simulink model "mtv1_with_slosh"  (R2014b)
settings: Solver=ode4  SolverMode=SingleTasking  StartTime=0.0  StopTime=sim_stop_time  FixedStep=sim_time_step_size  RelTol=1e-3
PreLoadFcn:
  | nimbus_bus_all;
  | mtv_bus_all;
undefined symbols (not defined in the file or in its folder): csc_egt_egc_thruster, csc_egt_egc_thruster_lib, csc_eom_six_dof_integration_fwdeuler, csc_eom_six_dof_integration_lib, csc_rigid_body_dynamics, csc_rigid_body_dynamics_lib, csc_sim_mtv_simulation, csc_sim_mtv_simulation_lib, csc_thl_thrusters_mtv, csc_thl_thrusters_mtv_lib, csci_gsse_mtv, csci_gsse_mtv_lib, csu_rrk_rotational_kinematics, csu_rrk_rotational_kinematics_lib, csu_rtk_translational_kinematics, csu_rtk_translational_kinematics_lib, csu_tpl_thruster_propellant_mtv, csu_tpl_thruster_propellant_mtv_lib, egt_feed_pressure, egt_g_times_isp, egt_pc_to_thrust_offset, egt_pc_to_thrust_slope, ini_epoch_seconds, ini_landed_flag, ini_thrust_to_weight_takeoff_limit, mpl_gn2_mass_initial, mpl_htp_mass_initial, sim_time_step_size, swm_num_switches, tpl_coarse_acs_thrust_to_isp, tpl_egc_chamber_pressure_to_thrust, tpl_egc_throttle_to_mdot_gain, tpl_egc_throttle_to_thrust, tpl_egc_throttle_to_thrust_gain
libraries: util_common_lib x13, util_info_lib x10, simulink x8, csu_spv_simulated_press_valves_lib x4, util_quat_lib x3, util_event_lib x2, util_frame_rotation_lib x2, csci_fsw_mtv_lib x1, csc_gnd_sta_lib x1, telem_conversion_lib x1, util_thruster_lib x1, csc_enf_environmental_forces_mtv_lib x1
(part 1 of 2)
settings Model: ExtModeTrigDuration=100  Creator=ianmga  LastModifiedBy=mstewart
settings DataIOCC: LimitDataPoints=off  SaveOutput=off  SaveTime=off  StateSaveName=tmp_raccel_xout  SignalLoggingName=raw_event_logs
settings OptimizationCC: ExpressionDepthLimit=2147483647  InitFltsAndDblsToZero=on  OptimizeModelRefInitCode=on
settings DebuggingCC: CheckSSInitialOutputMsg=off  UnderspecifiedInitializationDetection=Classic  MergeDetectMultiDrivingBlocksExec=none  UnderSpecifiedDataTypeMsg=warning  FcnCallInpInsideContextMsg=UseLocalSettings  BusObjectLabelMismatch=error  StateNameClashWarn=warning  StrictBusMsg=WarnOnBusTreatedAsVector
settings HardwareCC: TargetHWDeviceType=32-bit Generic
settings SFSimCC: SimParseCustomCode=off
settings SFSimCC: SimUserIncludeDirs=|
  | ../sim/fhw/sensors/cameras/kir
  | ../fsw/est/kcv
  | ../fsw/est/kfd
  | ../externals/minopencv/include
settings RTWCC: SystemTargetFile=ert.tlc  GenCodeOnly=on  TemplateMakefile=ert_default_tmf  Description=Embedded Coder  RetainRTWFile=on  ProcessScript=ert_make_rtw_hook  RTWUseSimCustomCode=on
settings RTWCC: CustomInclude=|
  | ../sim/fhw/sensors/cameras/kir
  | ../fsw/est/kcv
  | ../fsw/est/kfd
  | ../externals/minopencv/include
settings CodeAppCC: ForceParamTrailComments=on  IgnoreCustomStorageClasses=off  MaxIdLength=128  SimulinkDataObjDesc=on  SFDataObjDesc=on  MangleLength=10  CustomSymbolStrType=$N$R$M  InsertBlockDesc=on  InternalIdentifier=Classic  ReqsInCode=on
settings ERTTargetCC: GenerateSampleERTMain=on  MultiInstanceERTCode=on  CodeInterfacePackaging=Reusable function  RootIOFormat=Structure reference  ERTCustomFileTemplate=csl_interface.tlc

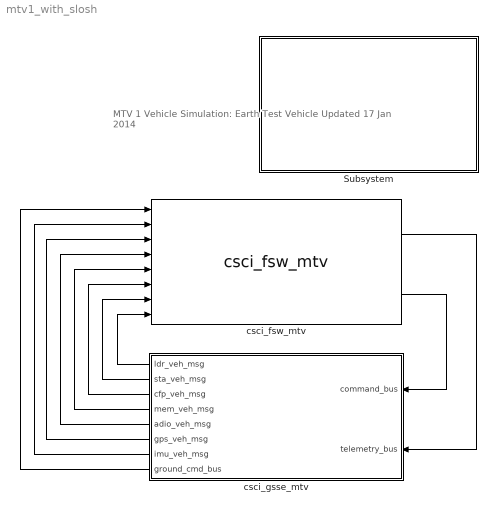
== system mtv1_with_slosh ==
  note: MTV 1 Vehicle Simulation: Earth Test Vehicle
      |
      | Updated 17 Jan 2014
  Subsystem : Subsystem
      mask Display: image('nimbus2.png')
  csci_fsw_mtv : csci_fsw_mtv_lib/csci_fsw_mtv
  csci_gsse_mtv : Subsystem  AncestorBlock=csci_gsse_mtv_lib/csci_gsse_mtv
  wires:
  csci_fsw_mtv/1 -> csci_gsse_mtv/2(telemetry_bus)
  csci_gsse_mtv/2(sta_veh_msg) -> csci_fsw_mtv/7
  csci_fsw_mtv/2 -> csci_gsse_mtv/1(command_bus)
  csci_gsse_mtv/1(ldr_veh_msg) -> csci_fsw_mtv/8
  csci_gsse_mtv/3(cfp_veh_msg) -> csci_fsw_mtv/6
  csci_gsse_mtv/4(mem_veh_msg) -> csci_fsw_mtv/5
  csci_gsse_mtv/5(adio_veh_msg) -> csci_fsw_mtv/4
  csci_gsse_mtv/6(gps_veh_msg) -> csci_fsw_mtv/3
  csci_gsse_mtv/8(ground_cmd_bus) -> csci_fsw_mtv/1
  csci_gsse_mtv/7(imu_veh_msg) -> csci_fsw_mtv/2

== system mtv1_with_slosh/Subsystem ==

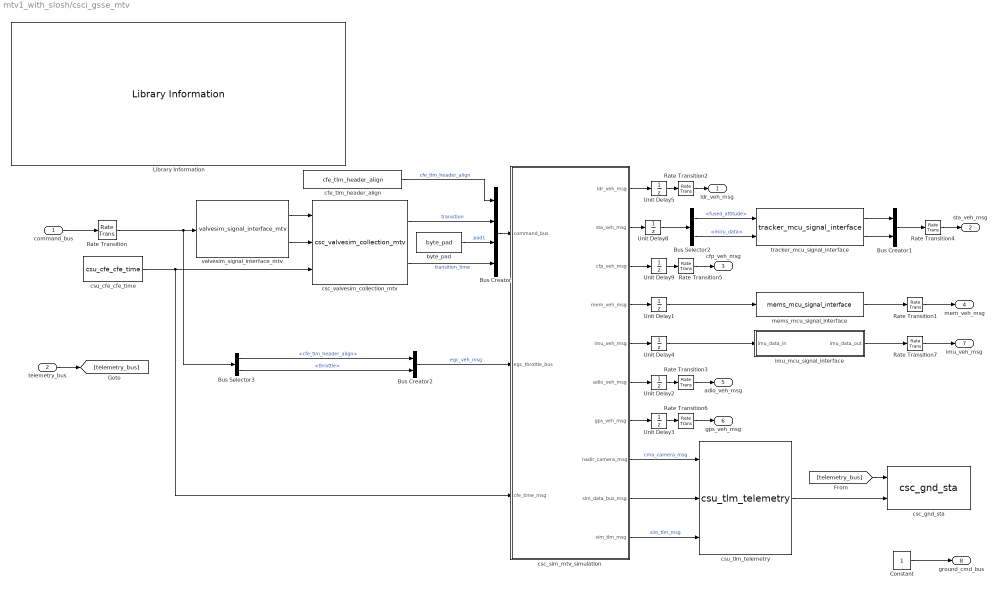
== system mtv1_with_slosh/csci_gsse_mtv ==
  command_bus : Inport
  telemetry_bus : Inport  Port=2
  Bus Creator : BusCreator  OutDataTypeStr=Bus: thr_sim_msg  NonVirtualBus=on
  Bus Creator2 : BusCreator  Inputs=2  OutDataTypeStr=Bus: egc_veh_msg  NonVirtualBus=on
  Bus Selector2 : BusSelector  OutputSignals=fused_attitude,miru_data
  Bus Selector3 : BusSelector  OutputSignals=egc_bus_msg.cfe_tlm_header_align,egc_bus_msg.throttle
  Bus Creator1 : BusCreator  Inputs=2
  Constant : Constant
  Library Information : util_info_lib/Library Information  owner='NONE'
  Rate Transition{,1..7} (8 alike) : RateTransition  Integrity=off
  Unit Delay{1..5,8..9} (7 alike) : UnitDelay  SampleTime=-1
  byte_pad : util_common_lib/byte_pad  n_bytes=6
  cfe_tlm_header_align : util_common_lib/cfe_tlm_header_align
  csc_gnd_sta : csc_gnd_sta_lib/csc_gnd_sta  dir_name=scenario_data_dir
  csc_sim_mtv_simulation : Subsystem  Tag=GSSE; MDL_TICK=THR_SIM_MSG  AncestorBlock=csc_sim_mtv_simulation_lib/csc_sim_mtv_simulation  TreatAsAtomicUnit=on
  csc_valvesim_collection_mtv : csc_valvesim_collection_mtv_lib/csc_valvesim_collection_mtv  SystemSampleTime=-1
  csu_cfe_cfe_time : csu_cfe_cfe_time_lib/csu_cfe_cfe_time  sch_dt=sim_time_step_size
  csu_tlm_telemetry : csu_tlm_telemetry_lib/csu_tlm_telemetry  num_inputs=3  output_bus_name=sim_telemetry_bus_msg
  imu_mcu_signal_interface : Subsystem
  mems_mcu_signal_interface : csu_mems_mcu_signal_interface_lib/mems_mcu_signal_interface
  tracker_mcu_signal_interface : csu_tracker_mcu_signal_interface_lib/tracker_mcu_signal_interface
  valvesim_signal_interface_mtv : csu_valvesim_signal_interface_mtv_lib/valvesim_signal_interface_mtv
  ldr_veh_msg : Outport
  sta_veh_msg : Outport  Port=2
  cfp_veh_msg : Outport  Port=3
  mem_veh_msg : Outport  Port=4
  adio_veh_msg : Outport  Port=5
  gps_veh_msg : Outport  Port=6
  imu_veh_msg : Outport  Port=7
  ground_cmd_bus : Outport  Port=8
  wires:
  telemetry_bus/1 -> [telemetry_bus]
  csc_sim_mtv_simulation/9(sim_data_bus_msg) -> csu_tlm_telemetry/2
  Unit Delay9/1 -> Rate Transition5/1
  Unit Delay5/1 -> Rate Transition2/1
  csc_sim_mtv_simulation/1(ldr_veh_msg) -> Unit Delay5/1
  csc_sim_mtv_simulation/3(cfp_veh_msg) -> Unit Delay9/1
  Constant/1 -> ground_cmd_bus/1
  command_bus/1 -> Rate Transition/1
  Rate Transition2/1 -> ldr_veh_msg/1
  Rate Transition4/1 -> sta_veh_msg/1
  Rate Transition5/1 -> cfp_veh_msg/1
  csc_sim_mtv_simulation/2(sta_veh_msg) -> Unit Delay8/1
  csc_sim_mtv_simulation/8(nadir_camera_msg) -> csu_tlm_telemetry/1  "cma_camera_msg"
  csc_sim_mtv_simulation/10(sim_tlm_msg) -> csu_tlm_telemetry/3  "sim_tlm_msg"
  csu_tlm_telemetry/1 -> csc_gnd_sta/2
  [telemetry_bus] -> csc_gnd_sta/1
  valvesim_signal_interface_mtv/1 -> csc_valvesim_collection_mtv/1
  csc_valvesim_collection_mtv/1 -> Bus Creator/2  "transition"
  csc_valvesim_collection_mtv/2 -> Bus Creator/4  "transition_time"
  Bus Creator/1 -> csc_sim_mtv_simulation/1(command_bus)
  csu_cfe_cfe_time/1 -> csc_sim_mtv_simulation/3(cfe_time_msg), csc_valvesim_collection_mtv/3
  byte_pad/1 -> Bus Creator/3  "pad1"
  Rate Transition/1 -> Bus Selector3/1, valvesim_signal_interface_mtv/1
  Bus Creator2/1 -> csc_sim_mtv_simulation/2(egc_throttle_bus)  "egc_veh_msg"
  cfe_tlm_header_align/1 -> Bus Creator/1  "cfe_tlm_header_align"
  valvesim_signal_interface_mtv/2 -> csc_valvesim_collection_mtv/2
  Bus Creator1/1 -> Rate Transition4/1
  tracker_mcu_signal_interface/2 -> Bus Creator1/2
  tracker_mcu_signal_interface/1 -> Bus Creator1/1
  Bus Selector2/2 -> tracker_mcu_signal_interface/2  "<miru_data>"
  Bus Selector2/1 -> tracker_mcu_signal_interface/1  "<fused_attitude>"
  Unit Delay8/1 -> Bus Selector2/1
  csc_sim_mtv_simulation/4(mem_veh_msg) -> Unit Delay1/1
  Unit Delay1/1 -> mems_mcu_signal_interface/1
  Rate Transition1/1 -> mem_veh_msg/1
  mems_mcu_signal_interface/1 -> Rate Transition1/1
  Bus Selector3/1 -> Bus Creator2/1  "<cfe_tlm_header_align>"
  Bus Selector3/2 -> Bus Creator2/2  "<throttle>"
  Unit Delay2/1 -> Rate Transition3/1
  csc_sim_mtv_simulation/6(adio_veh_msg) -> Unit Delay2/1
  Rate Transition3/1 -> adio_veh_msg/1
  Unit Delay3/1 -> Rate Transition6/1
  Rate Transition6/1 -> gps_veh_msg/1
  csc_sim_mtv_simulation/7(gps_veh_msg) -> Unit Delay3/1
  csc_sim_mtv_simulation/5(imu_veh_msg) -> Unit Delay4/1
  Unit Delay4/1 -> imu_mcu_signal_interface/1(imu_data_in)
  Rate Transition7/1 -> imu_veh_msg/1
  imu_mcu_signal_interface/1(imu_data_out) -> Rate Transition7/1

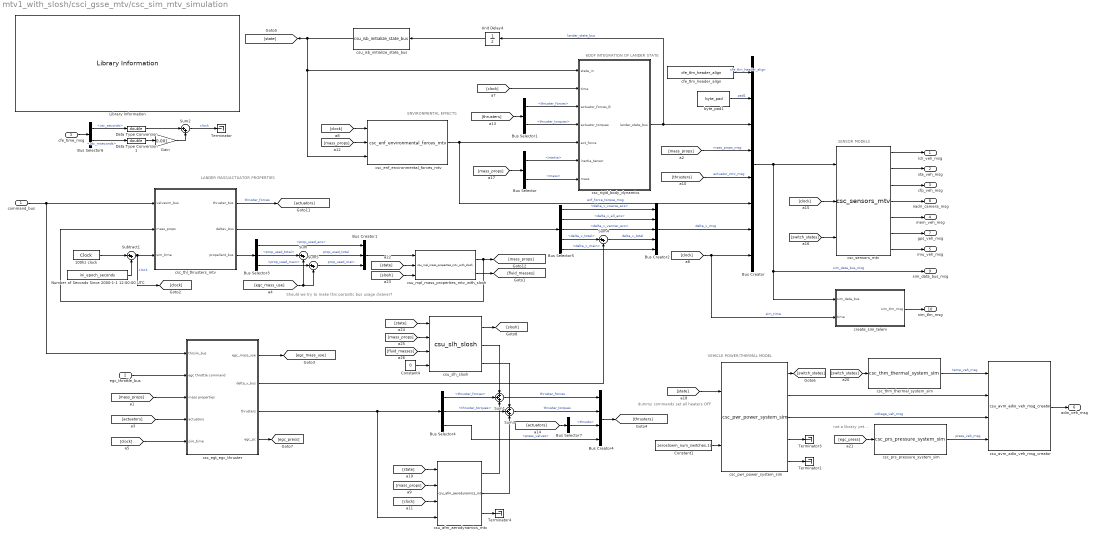
== system mtv1_with_slosh/csci_gsse_mtv/csc_sim_mtv_simulation ==
  note: not a library yet....
  note: VEHICLE POWER/THERMAL MODEL
  note: dummy commands set all heaters OFF
  note: LANDER MASS/ACTUATOR PROPERTIES
  note: 6DOF INTEGRATION OF LANDER STATE
  note: ENVIRONMENTAL EFFECTS
  note: SENSOR MODELS
  note: Should we try to make this parasitic bus usage cleaner?
  command_bus : Inport
  egc_throttle_bus : Inport  Port=2
  cfe_time_msg : Inport  Port=3  OutDataTypeStr=Bus: cfe_time_msg
  100hz clock : DigitalClock  SampleTime=sim_time_step_size
  Bus Creator : BusCreator  Inputs=8  OutDataTypeStr=Bus: sim_data_mtv_msg  NonVirtualBus=on
  Bus Creator1 : BusCreator  Inputs=3
  Bus Creator2 : BusCreator  Inputs=5
  Bus Creator4 : BusCreator  OutDataTypeStr=Bus: actuator_mtv_msg_t
  Bus Selector : BusSelector  OutputSignals=inertia,mass
  Bus Selector1 : BusSelector  OutputSignals=thruster_forces,thruster_torques
  Bus Selector3 : BusSelector  OutputSignals=prop_used_acs,prop_used_total,prop_used_main
  Bus Selector4 : BusSelector  OutputSignals=thruster_forces,thruster_torques,press_valves
  Bus Selector5 : BusSelector  OutputSignals=delta_v_coarse_acs,delta_v_all_acs,delta_v_vernier_acs,delta_v_total,delta_v_main
  Bus Selector6 : BusSelector  OutputSignals=utc_seconds,utc_mseconds
  Bus Selector7 : BusSelector  OutputSignals=thrusts
  Constant1 : Constant  Value=zeros(swm_num_switches,1)  OutDataTypeStr=double
  Constant4 : Constant  Value=0
  Data Type Conversion : DataTypeConversion  OutDataTypeStr=double
  Data Type Conversion1 : DataTypeConversion  OutDataTypeStr=double
  Gain : Gain  Gain=0.001
  Library Information : util_info_lib/Library Information  owner='NONE'
  Number of Seconds Since 2000-1-1 12:00:00 UTC : Constant  Description=|  Value=ini_epoch_seconds
      | Number of Seconds                   
      | July 4, 2014 22:40:00 UTC           
      | Calculate on Web Site:              
      | www.mbari.org/staff/rich/utccalc.htm
  Subtract1 : Sum  Inputs=|++
  Sum{,2,4..5} (4 alike) : Sum  Inputs=|++
  Sum1 : Sum  Inputs=+++
  Sum3 : Sum  Inputs=+++
  Terminator{,1,3..4} (4 alike) : Terminator
  Unit Delay4 : UnitDelay  SampleTime=-1
  byte_pad1 : util_common_lib/byte_pad  n_bytes=4
  cfe_tlm_header_align : util_common_lib/cfe_tlm_header_align
  create_sim_telem : Subsystem
  csc_egt_egc_thruster : Subsystem  AncestorBlock=csc_egt_egc_thruster_lib/csc_egt_egc_thruster
  csc_enf_environmental_forces_mtv : csc_enf_environmental_forces_mtv_lib/csc_enf_environmental_forces_mtv
  csc_prs_pressure_system_sim : csc_prs_pressure_system_sim_lib/csc_prs_pressure_system_sim
  csc_pwr_power_system_sim : csc_pwr_power_system_sim_lib/csc_pwr_power_system_sim
  csc_rigid_body_dynamics : Subsystem  AncestorBlock=csc_rigid_body_dynamics_lib/csc_rigid_body_dynamics
  csc_sensors_mtv : csc_sensors_mtv_lib/csc_sensors_mtv
  csc_thl_thrusters_mtv : Subsystem  AncestorBlock=csc_thl_thrusters_mtv_lib/csc_thl_thrusters_mtv
  csc_thm_thermal_system_sim : csc_thm_thermal_system_sim_lib/csc_thm_thermal_system_sim
  csu_afm_aerodynamics_mtv : csu_afm_aerodynamics_lib/csu_afm_aerodynamics_mtv  SystemSampleTime=-1
  csu_avm_adio_veh_msg_creator : csu_avm_adio_veh_msg_creator_lib/csu_avm_adio_veh_msg_creator
  csu_isb_initialize_state_bus : csu_isb_initialize_state_bus_lib/csu_isb_initialize_state_bus
  csu_mpl_mass_properties_mtv_with_slosh : csu_mpl_mass_properties_mtv_lib/csu_mpl_mass_properties_mtv_with_slosh
  csu_slh_slosh : csu_slh_slosh/csu_slh_slosh
  ldr_veh_msg : Outport
  sta_veh_msg : Outport  Port=2
  cfp_veh_msg : Outport  Port=3
  mem_veh_msg : Outport  Port=4
  imu_veh_msg : Outport  Port=5
  adio_veh_msg : Outport  Port=6
  gps_veh_msg : Outport  Port=7
  nadir_camera_msg : Outport  Port=8
  sim_data_bus_msg : Outport  Port=9
  sim_tlm_msg : Outport  Port=10
  wires:
  csu_afm_aerodynamics_mtv/3 -> Terminator4/1
  [clock] -> csu_afm_aerodynamics_mtv/3
  csu_afm_aerodynamics_mtv/2 -> Sum3/3
  Sum3/1 -> Bus Creator4/2  "thruster_torques"
  csu_afm_aerodynamics_mtv/1 -> Sum1/3
  Bus Selector7/1 -> Bus Creator4/3  "<thrusts>"
  [actuators] -> Bus Selector7/1
  Bus Creator4/1 -> [thrusters]
  Sum1/1 -> Bus Creator4/1  "thruster_forces"
  Bus Selector4/1 -> Sum1/2  "<thruster_forces>"
  Bus Selector4/2 -> Sum3/2  "<thruster_torques>"
  csc_egt_egc_thruster/3(thrusters) -> csu_afm_aerodynamics_mtv/4, Bus Selector4/1
  [switch_states] -> csc_sensors_mtv/3
  csc_pwr_power_system_sim/5 -> Terminator1/1
  csc_pwr_power_system_sim/4 -> Terminator3/1
  csc_pwr_power_system_sim/1 -> [switch_states]
  [state] -> csc_pwr_power_system_sim/1
  Constant1/1 -> csc_pwr_power_system_sim/2
  [clock] -> csc_sensors_mtv/2
  Unit Delay4/1 -> csu_isb_initialize_state_bus/1
  csu_isb_initialize_state_bus/1 -> csc_enf_environmental_forces_mtv/3, csc_rigid_body_dynamics/1(state_in), [state]
  [clock] -> csc_rigid_body_dynamics/2(time)
  cfe_tlm_header_align/1 -> Bus Creator/1  "cfe_tlm_header_align"
  csc_sensors_mtv/4 -> nadir_camera_msg/1
  csc_sensors_mtv/3 -> cfp_veh_msg/1
  csc_sensors_mtv/2 -> sta_veh_msg/1
  csc_sensors_mtv/1 -> ldr_veh_msg/1
  Bus Selector6/1 -> Data Type Conversion/1  "<utc_seconds>"
  Gain/1 -> Sum2/2
  Data Type Conversion1/1 -> Gain/1
  Data Type Conversion/1 -> Sum2/1
  Bus Selector6/2 -> Data Type Conversion1/1  "<utc_mseconds>"
  cfe_time_msg/1 -> Bus Selector6/1
  egc_throttle_bus/1 -> csc_egt_egc_thruster/2(egc throttle command)
  [mass_props] -> csc_egt_egc_thruster/3(mass properties)
  [actuators] -> csc_egt_egc_thruster/4(actuators)
  Bus Selector5/1 -> Bus Creator2/1  "<delta_v_coarse_acs>"
  Bus Selector5/2 -> Bus Creator2/2  "<delta_v_all_acs>"
  Bus Selector5/3 -> Bus Creator2/3  "<delta_v_vernier_acs>"
  Bus Selector5/5 -> Bus Creator2/5  "<delta_v_main>"
  Sum4/1 -> Bus Creator2/4  "delta_v_total"
  Bus Selector5/4 -> Sum4/1  "<delta_v_total>"
  csc_thl_thrusters_mtv/2(deltav_bus) -> Bus Selector5/1
  Bus Creator2/1 -> Bus Creator/7  "delta_v_msg"
  csc_egt_egc_thruster/2(delta_v_bus) -> Sum4/2
  Bus Selector3/3 -> Sum5/1  "<prop_used_main>"
  Bus Selector3/1 -> Bus Creator1/1  "<prop_used_acs>"
  Sum/1 -> Bus Creator1/2  "prop_used_total"
  [egc_mass_use] -> Sum5/2, Sum/2
  Bus Selector3/2 -> Sum/1  "<prop_used_total>"
  csc_egt_egc_thruster/1(egc_mass_use) -> [egc_mass_use]
  csc_thl_thrusters_mtv/3(propellant_bus) -> Bus Selector3/1
  byte_pad1/1 -> Bus Creator/2  "pad1"
  Subtract1/1 -> [clock], csc_thl_thrusters_mtv/3(sim_time)  "clock"
  [clock] -> Bus Creator/8, create_sim_telem/2(time)  "sim_time"
  create_sim_telem/1(sim_tlm_msg) -> sim_tlm_msg/1
  Bus Creator/1 -> create_sim_telem/1(sim_data_bus), sim_data_bus_msg/1, csc_sensors_mtv/1  "sim_data_bus_msg"
  csc_rigid_body_dynamics/1(lander_state_bus) -> Unit Delay4/1, Bus Creator/3  "lander_state_bus"
  [mass_props] -> Bus Selector/1
  [thrusters] -> Bus Selector1/1
  [thrusters] -> Bus Creator/5  "actuator_mtv_msg"
  [mass_props] -> Bus Creator/4  "mass_props_msg"
  Bus Selector/2 -> csc_rigid_body_dynamics/7(mass)  "<mass>"
  Bus Selector/1 -> csc_rigid_body_dynamics/6(inertia_tensor)  "<inertia>"
  Bus Selector1/1 -> csc_rigid_body_dynamics/3(actuator_forces_B)  "<thruster_forces>"
  Bus Selector1/2 -> csc_rigid_body_dynamics/4(actuator_torques)  "<thruster_torques>"
  csc_enf_environmental_forces_mtv/1 -> csc_rigid_body_dynamics/5(ext_force), Bus Creator/6  "enf_force_torque_msg"
  csc_thl_thrusters_mtv/1(thruster_bus) -> [actuators]  "thruster_forces"
  [clock] -> csc_enf_environmental_forces_mtv/1
  [mass_props] -> csc_enf_environmental_forces_mtv/2
  csc_sensors_mtv/5 -> mem_veh_msg/1
  Number of Seconds Since 2000-1-1 12:00:00 UTC/1 -> Subtract1/2
  100hz clock/1 -> Subtract1/1
  Sum2/1 -> Terminator/1  "clock"
  [switch_states] -> csc_thm_thermal_system_sim/1
  csu_avm_adio_veh_msg_creator/1 -> adio_veh_msg/1
  csc_thm_thermal_system_sim/1 -> csu_avm_adio_veh_msg_creator/1  "temp_veh_msg"
  csc_pwr_power_system_sim/2 -> csu_avm_adio_veh_msg_creator/2
  csc_pwr_power_system_sim/3 -> csu_avm_adio_veh_msg_creator/3  "voltage_veh_msg"
  [egc_press] -> csc_prs_pressure_system_sim/1
  csc_prs_pressure_system_sim/1 -> csu_avm_adio_veh_msg_creator/4  "press_veh_msg"
  csc_egt_egc_thruster/4(egc_pc) -> [egc_press]
  command_bus/1 -> csc_egt_egc_thruster/1(thrsim_bus), csc_thl_thrusters_mtv/1(valvesim_bus)
  [clock] -> csc_egt_egc_thruster/5(sim_time)
  Sum5/1 -> Bus Creator1/3  "prop_used_main"
  Bus Selector4/3 -> Bus Creator4/4  "<press_valves>"
  csc_sensors_mtv/6 -> gps_veh_msg/1
  csc_sensors_mtv/7 -> imu_veh_msg/1
  [mass_props] -> csu_afm_aerodynamics_mtv/2
  [state] -> csu_afm_aerodynamics_mtv/1
  Bus Creator1/1 -> csu_mpl_mass_properties_mtv_with_slosh/1
  csu_mpl_mass_properties_mtv_with_slosh/1 -> [mass_props], csc_thl_thrusters_mtv/2(mass_props)
  csu_mpl_mass_properties_mtv_with_slosh/2 -> [fluid_masses]
  [state] -> csu_mpl_mass_properties_mtv_with_slosh/2
  [state] -> csu_slh_slosh/1
  [mass_props] -> csu_slh_slosh/2
  [fluid_masses] -> csu_slh_slosh/3
  Constant4/1 -> csu_slh_slosh/4
  csu_slh_slosh/3 -> Sum3/1
  csu_slh_slosh/2 -> Sum1/1
  csu_slh_slosh/1 -> [slosh]
  [slosh] -> csu_mpl_mass_properties_mtv_with_slosh/3

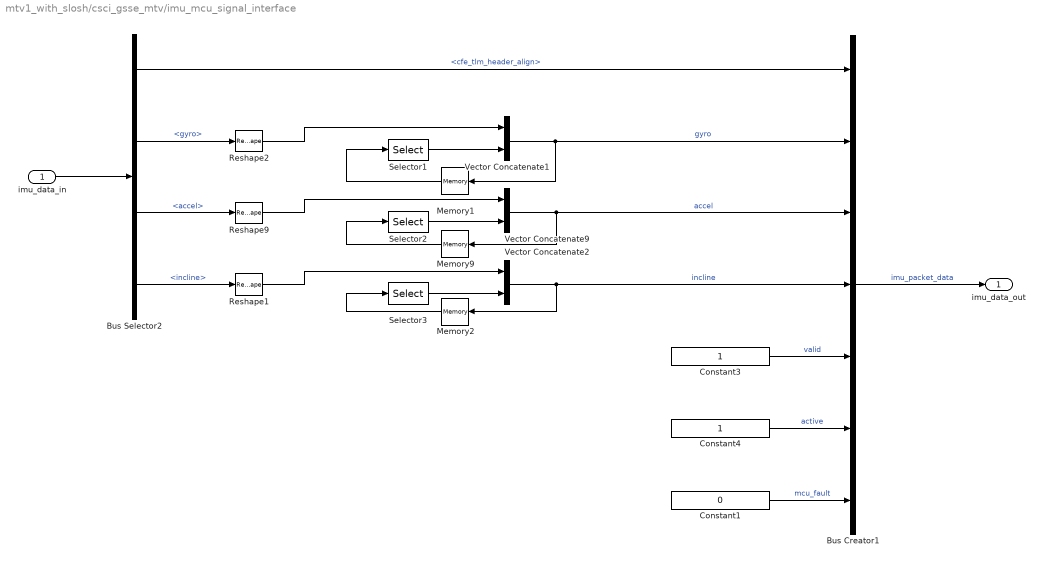
== system mtv1_with_slosh/csci_gsse_mtv/imu_mcu_signal_interface ==
  imu_data_in : Inport
  Bus Selector2 : BusSelector  OutputSignals=cfe_tlm_header_align,gyro,accel,incline
  Bus Creator1 : BusCreator  Inputs=7
  Constant1 : Constant  Value=0  OutDataTypeStr=uint8
  Constant3 : Constant  OutDataTypeStr=uint16
  Constant4 : Constant  OutDataTypeStr=uint8
  Memory1 : Memory  X0=zeros(10,3)  InheritSampleTime=on
  Memory2 : Memory  X0=zeros(10,3)  InheritSampleTime=on
  Memory9 : Memory  X0=zeros(10,3)  InheritSampleTime=on
  Reshape1 : Reshape  OutputDimensionality=Row vector (2-D)
  Reshape2 : Reshape  OutputDimensionality=Row vector (2-D)
  Reshape9 : Reshape  OutputDimensionality=Row vector (2-D)
  Selector1 : Selector  NumberOfDimensions=2  InputPortWidth=10  IndexOptions=Index vector (dialog),Select all  Indices=[1:9],1  OutputSizes=1,1
  Selector2 : Selector  NumberOfDimensions=2  InputPortWidth=10  IndexOptions=Index vector (dialog),Select all  Indices=[1:9],1  OutputSizes=1,1
  Selector3 : Selector  NumberOfDimensions=2  InputPortWidth=10  IndexOptions=Index vector (dialog),Select all  Indices=[1:9],1  OutputSizes=1,1
  Vector Concatenate1 : Concatenate  Mode=Multidimensional array
  Vector Concatenate2 : Concatenate  Mode=Multidimensional array
  Vector Concatenate9 : Concatenate  Mode=Multidimensional array
  imu_data_out : Outport
  wires:
  Bus Selector2/4 -> Reshape1/1  "<incline>"
  Memory2/1 -> Selector3/1
  Selector3/1 -> Vector Concatenate2/2
  Vector Concatenate2/1 -> Bus Creator1/4, Memory2/1  "incline"
  Reshape1/1 -> Vector Concatenate2/1
  Bus Selector2/1 -> Bus Creator1/1  "<cfe_tlm_header_align>"
  Bus Creator1/1 -> imu_data_out/1  "imu_packet_data"
  imu_data_in/1 -> Bus Selector2/1
  Memory1/1 -> Selector1/1
  Selector1/1 -> Vector Concatenate1/2
  Vector Concatenate1/1 -> Memory1/1, Bus Creator1/2  "gyro"
  Reshape2/1 -> Vector Concatenate1/1
  Memory9/1 -> Selector2/1
  Selector2/1 -> Vector Concatenate9/2
  Vector Concatenate9/1 -> Bus Creator1/3, Memory9/1  "accel"
  Reshape9/1 -> Vector Concatenate9/1
  Constant3/1 -> Bus Creator1/5  "valid"
  Constant4/1 -> Bus Creator1/6  "active"
  Constant1/1 -> Bus Creator1/7  "mcu_fault"
  Bus Selector2/2 -> Reshape2/1  "<gyro>"
  Bus Selector2/3 -> Reshape9/1  "<accel>"

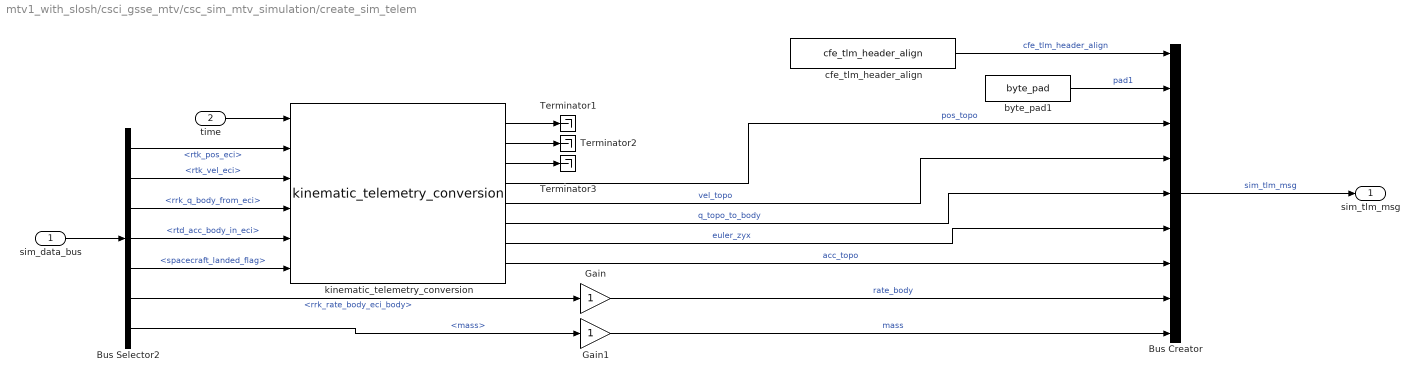
== system mtv1_with_slosh/csci_gsse_mtv/csc_sim_mtv_simulation/create_sim_telem ==
  sim_data_bus : Inport
  time : Inport  Port=2
  Bus Creator : BusCreator  Inputs=9  OutDataTypeStr=Bus: sim_tlm_msg  NonVirtualBus=on
  Bus Selector2 : BusSelector  OutputSignals=lander_state_bus.rtk_pos_eci,lander_state_bus.rtk_vel_eci,lander_state_bus.rrk_q_body_from_eci,lander_state_bus.rtd_acc_body_in_eci,lander_state_bus.spacecraft_landed_flag,lander_state_bus.rrk_rate_body_eci_body,mass_props_msg.mass
  Gain : Gain
  Gain1 : Gain
  Terminator1 : Terminator
  Terminator2 : Terminator
  Terminator3 : Terminator
  byte_pad1 : util_common_lib/byte_pad  n_bytes=4
  cfe_tlm_header_align : util_common_lib/cfe_tlm_header_align
  kinematic_telemetry_conversion : telem_conversion_lib/kinematic_telemetry_conversion
  sim_tlm_msg : Outport
  wires:
  cfe_tlm_header_align/1 -> Bus Creator/1  "cfe_tlm_header_align"
  byte_pad1/1 -> Bus Creator/2  "pad1"
  kinematic_telemetry_conversion/3 -> Terminator3/1
  kinematic_telemetry_conversion/2 -> Terminator2/1
  kinematic_telemetry_conversion/1 -> Terminator1/1
  Bus Creator/1 -> sim_tlm_msg/1  "sim_tlm_msg"
  kinematic_telemetry_conversion/8 -> Bus Creator/7  "acc_topo"
  kinematic_telemetry_conversion/7 -> Bus Creator/6  "euler_zyx"
  kinematic_telemetry_conversion/6 -> Bus Creator/5  "q_topo_to_body"
  kinematic_telemetry_conversion/5 -> Bus Creator/4  "vel_topo"
  sim_data_bus/1 -> Bus Selector2/1
  time/1 -> kinematic_telemetry_conversion/1
  Bus Selector2/1 -> kinematic_telemetry_conversion/2  "<rtk_pos_eci>"
  Bus Selector2/2 -> kinematic_telemetry_conversion/3  "<rtk_vel_eci>"
  Bus Selector2/3 -> kinematic_telemetry_conversion/4  "<rrk_q_body_from_eci>"
  Bus Selector2/4 -> kinematic_telemetry_conversion/5  "<rtd_acc_body_in_eci>"
  Bus Selector2/6 -> Gain/1  "<rrk_rate_body_eci_body>"
  Gain/1 -> Bus Creator/8  "rate_body"
  Bus Selector2/7 -> Gain1/1  "<mass>"
  Gain1/1 -> Bus Creator/9  "mass"
  kinematic_telemetry_conversion/4 -> Bus Creator/3  "pos_topo"
  Bus Selector2/5 -> kinematic_telemetry_conversion/6  "<spacecraft_landed_flag>"

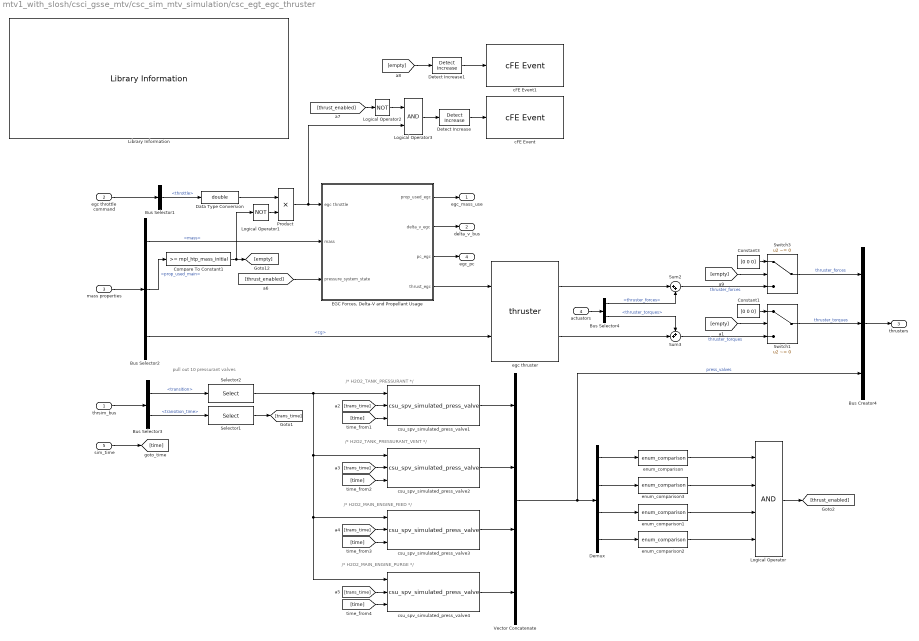
== system mtv1_with_slosh/csci_gsse_mtv/csc_sim_mtv_simulation/csc_egt_egc_thruster ==
  note: /* H2O2_MAIN_ENGINE_PURGE */
  note: /* H2O2_MAIN_ENGINE_FEED */
  note: /* H2O2_TANK_PRESSURANT_VENT */
  note: /* H2O2_TANK_PRESSURANT */
  note: pull out 10 pressurant valves
  thrsim_bus : Inport
  egc throttle command : Inport  Port=2
  mass properties : Inport  Port=3
  actuators : Inport  Port=4
  sim_time : Inport  Port=5
  Bus Creator4 : BusCreator  Inputs=3
  Bus Selector1 : BusSelector  OutputSignals=throttle
  Bus Selector2 : BusSelector  OutputSignals=mass,prop_used_main,cg
  Bus Selector3 : BusSelector  OutputSignals=transition,transition_time
  Bus Selector4 : BusSelector  OutputSignals=thruster_forces,thruster_torques
  Compare To Constant1 : simulink/Logic and Bit Operations/Compare To Constant  relop=>=  const=mpl_htp_mass_initial  OutDataTypeStr=boolean
  Constant1 : Constant  Value=[0 0 0]
  Constant3 : Constant  Value=[0 0 0]
  Data Type Conversion : DataTypeConversion  OutDataTypeStr=double
  Demux : Demux
  Detect Increase : simulink/Logic and Bit Operations/Detect Increase  vinit=0.0  InputProcessing=Inherited  OutDataTypeStr=boolean
  Detect Increase1 : simulink/Logic and Bit Operations/Detect Increase  vinit=0.0  InputProcessing=Inherited  OutDataTypeStr=boolean
  "EGC Forces, Delta-V and Propellant Usage" : Subsystem
  Library Information : util_info_lib/Library Information  owner='NONE'
  Logical Operator : Logic  Inputs=4  AllPortsSameDT=off  OutDataTypeStr=boolean
  Logical Operator1 : Logic  Operator=NOT  AllPortsSameDT=off  OutDataTypeStr=boolean
  Logical Operator2 : Logic  Operator=NOT  AllPortsSameDT=off  OutDataTypeStr=boolean
  Logical Operator3 : Logic  AllPortsSameDT=off  OutDataTypeStr=boolean
  Product : Product
  Selector1 : Selector  InputPortWidth=22  Indices=[13:22]
  Selector2 : Selector  InputPortWidth=22  Indices=[13:22]
  Sum2 : Sum  Inputs=|++
  Sum3 : Sum  Inputs=++|
  Switch1 : Switch  Criteria=u2 ~= 0
  Switch3 : Switch  Criteria=u2 ~= 0
  Vector Concatenate : Concatenate  NumInputs=4
  cFE Event : util_event_lib/cFE Event  event_message='EGC commanded with bad latch valve config. No thrust.'  event_id=22  event_severity=INFORMATION  event_use_enums=off  event_enum_types={}
  cFE Event1 : util_event_lib/cFE Event  event_message='Out of HTP!'  event_id=22  event_severity=INFORMATION  event_use_enums=off  event_enum_types={}
  csu_spv_simulated_press_valve1 : csu_spv_simulated_press_valves_lib/csu_spv_simulated_press_valve  thruster_idx=1  num_thrusters=10  energized_value=1  deenergized_value=0
  csu_spv_simulated_press_valve2 : csu_spv_simulated_press_valves_lib/csu_spv_simulated_press_valve  thruster_idx=2  num_thrusters=10  energized_value=0  deenergized_value=1
  csu_spv_simulated_press_valve3 : csu_spv_simulated_press_valves_lib/csu_spv_simulated_press_valve  thruster_idx=4  num_thrusters=10  energized_value=1  deenergized_value=0
  csu_spv_simulated_press_valve4 : csu_spv_simulated_press_valves_lib/csu_spv_simulated_press_valve  thruster_idx=5  num_thrusters=10  energized_value=1  deenergized_value=0
  egc thruster : util_thruster_lib/thruster  Thruster_Position=tfl_thruster_egc_position  Thruster_Orientation=tfl_thruster_egc_orientation
  enum_comparison{,1..3} (4 alike) : util_common_lib/enum_comparison  comparison_type===
  egc_mass_use : Outport
  delta_v_bus : Outport  Port=2
  thrusters : Outport  Port=3
  egc_pc : Outport  Port=4
  wires:
  "EGC Forces, Delta-V and Propellant Usage"/3(pc_egc) -> egc_pc/1
  Product/1 -> Logical Operator3/2, "EGC Forces, Delta-V and Propellant Usage"/1(egc throttle)
  Switch1/1 -> Bus Creator4/2  "thruster_torques"
  Switch3/1 -> Bus Creator4/1  "thruster_forces"
  Constant3/1 -> Switch3/1
  egc throttle command/1 -> Bus Selector1/1
  Data Type Conversion/1 -> Product/1
  Sum2/1 -> Switch3/3  "thruster_forces"
  Sum3/1 -> Switch1/3  "thruster_torques"
  Bus Creator4/1 -> thrusters/1
  Bus Selector4/2 -> Sum3/1  "<thruster_torques>"
  egc thruster/2 -> Sum3/2
  egc thruster/1 -> Sum2/1
  actuators/1 -> Bus Selector4/1
  Bus Selector4/1 -> Sum2/2  "<thruster_forces>"
  Bus Selector2/3 -> egc thruster/2  "<cg>"
  Bus Selector2/1 -> "EGC Forces, Delta-V and Propellant Usage"/2(mass)  "<mass>"
  mass properties/1 -> Bus Selector2/1
  "EGC Forces, Delta-V and Propellant Usage"/4(thrust_egc) -> egc thruster/1
  "EGC Forces, Delta-V and Propellant Usage"/2(delta_v_egc) -> delta_v_bus/1
  "EGC Forces, Delta-V and Propellant Usage"/1(prop_used_egc) -> egc_mass_use/1
  Bus Selector1/1 -> Data Type Conversion/1  "<throttle>"
  Constant1/1 -> Switch1/1
  Compare To Constant1/1 -> [empty], Logical Operator1/1
  [empty] -> Switch3/2
  [empty] -> Switch1/2
  thrsim_bus/1 -> Bus Selector3/1
  Selector1/1 -> [trans_time]
  Bus Selector3/1 -> Selector2/1  "<transition>"
  Bus Selector3/2 -> Selector1/1  "<transition_time>"
  [trans_time] -> csu_spv_simulated_press_valve1/2
  sim_time/1 -> [time]
  [time] -> csu_spv_simulated_press_valve1/3
  [trans_time] -> csu_spv_simulated_press_valve2/2
  [time] -> csu_spv_simulated_press_valve2/3
  [trans_time] -> csu_spv_simulated_press_valve3/2
  [time] -> csu_spv_simulated_press_valve3/3
  [trans_time] -> csu_spv_simulated_press_valve4/2
  [time] -> csu_spv_simulated_press_valve4/3
  Selector2/1 -> csu_spv_simulated_press_valve4/1, csu_spv_simulated_press_valve3/1, csu_spv_simulated_press_valve2/1, csu_spv_simulated_press_valve1/1
  csu_spv_simulated_press_valve1/1 -> Vector Concatenate/1
  csu_spv_simulated_press_valve3/1 -> Vector Concatenate/3
  csu_spv_simulated_press_valve4/1 -> Vector Concatenate/4
  csu_spv_simulated_press_valve2/1 -> Vector Concatenate/2
  enum_comparison/1 -> Logical Operator/1
  enum_comparison3/1 -> Logical Operator/2
  enum_comparison1/1 -> Logical Operator/3
  enum_comparison2/1 -> Logical Operator/4
  Logical Operator/1 -> [thrust_enabled]
  [thrust_enabled] -> "EGC Forces, Delta-V and Propellant Usage"/3(pressure_system_state)
  Bus Selector2/2 -> Compare To Constant1/1  "<prop_used_main>"
  Logical Operator1/1 -> Product/2
  Vector Concatenate/1 -> Bus Creator4/3, Demux/1  "press_valves"
  Demux/1 -> enum_comparison/1
  Demux/2 -> enum_comparison3/1
  Demux/3 -> enum_comparison1/1
  Demux/4 -> enum_comparison2/1
  Logical Operator3/1 -> Detect Increase/1
  Logical Operator2/1 -> Logical Operator3/1
  [thrust_enabled] -> Logical Operator2/1
  Detect Increase/1 -> cFE Event/1
  [empty] -> Detect Increase1/1
  Detect Increase1/1 -> cFE Event1/1

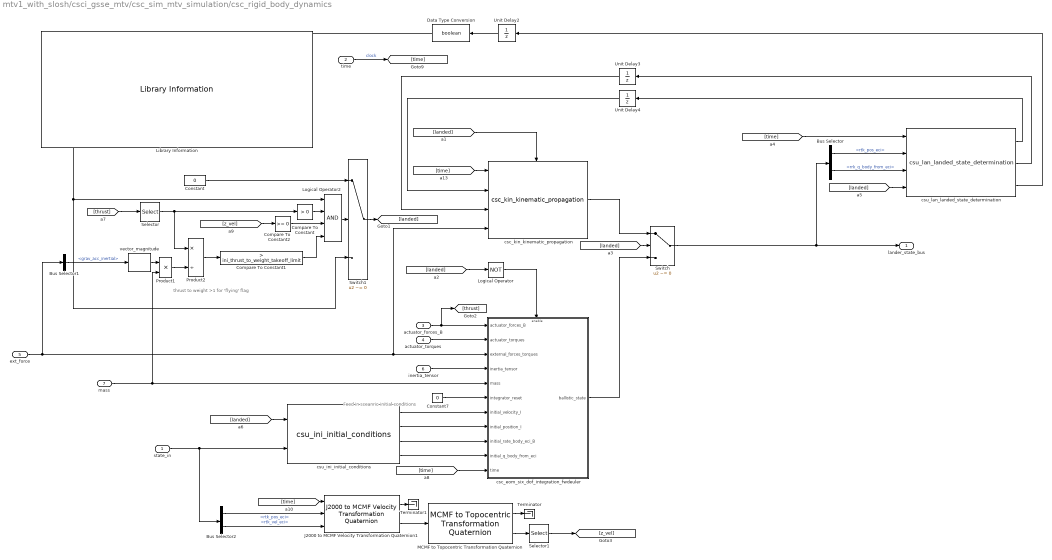
== system mtv1_with_slosh/csci_gsse_mtv/csc_sim_mtv_simulation/csc_rigid_body_dynamics ==
  note: thrust to weight >1 for
      | 'flying' flag
  note: Feed in sceanrio initial conditions
  state_in : Inport
  time : Inport  Port=2
  actuator_forces_B : Inport  Port=3
  actuator_torques : Inport  Port=4
  ext_force : Inport  Port=5
  inertia_tensor : Inport  Port=6
  mass : Inport  Port=7
  Bus Selector : BusSelector  OutputSignals=rtk_pos_eci,rrk_q_body_from_eci
  Bus Selector1 : BusSelector  OutputSignals=grav_acc_inertial
  Bus Selector2 : BusSelector  OutputSignals=rtk_pos_eci,rtk_vel_eci
  Compare To Constant : simulink/Logic and Bit Operations/Compare To Constant  relop=>  const=0  OutDataTypeStr=boolean
  Compare To Constant1 : simulink/Logic and Bit Operations/Compare To Constant  relop=>  const=ini_thrust_to_weight_takeoff_limit  OutDataTypeStr=boolean
  Compare To Constant2 : simulink/Logic and Bit Operations/Compare To Constant  relop=>=  const=0  OutDataTypeStr=boolean
  Constant : Constant  Value=0  OutDataTypeStr=boolean
  Constant7 : Constant  Value=0
  Data Type Conversion : DataTypeConversion  OutDataTypeStr=boolean
  J2000 to MCMF Velocity Transformation Quaternion1 : util_frame_rotation_lib/J2000 to MCMF Velocity Transformation Quaternion  SystemSampleTime=-1
  Library Information : util_info_lib/Library Information  owner='escrane'
  Logical Operator : Logic  Operator=NOT  AllPortsSameDT=off  OutDataTypeStr=boolean
  Logical Operator2 : Logic  Inputs=4  AllPortsSameDT=off  OutDataTypeStr=boolean
  MCMF to Topocentric Transformation Quaternion : util_frame_rotation_lib/MCMF to Topocentric  Transformation Quaternion  SystemSampleTime=-1
  Product1 : Product  RndMeth=Zero
  Product2 : Product  Inputs=*/  RndMeth=Zero
  Selector : Selector  InputPortWidth=3  Indices=3
  Selector1 : Selector  InputPortWidth=3  Indices=3
  Switch : Switch  Criteria=u2 ~= 0
  Switch1 : Switch  Criteria=u2 ~= 0
  Terminator : Terminator
  Terminator1 : Terminator
  Unit Delay2 : UnitDelay  InitialCondition=boolean(ini_landed_flag)  SampleTime=-1
  Unit Delay3 : UnitDelay  InitialCondition=[0 0 0 1]  SampleTime=-1
  Unit Delay4 : UnitDelay  InitialCondition=[0 0 0]  SampleTime=-1
  csc_eom_six_dof_integration_fwdeuler : Subsystem  AncestorBlock=csc_eom_six_dof_integration_lib/csc_eom_six_dof_integration_fwdeuler
  csc_kin_kinematic_propagation : csc_kin_kinematic_propagation_lib/csc_kin_kinematic_propagation
  csu_ini_initial_conditions : csu_ini_initial_conditions_lib/csu_ini_initial_conditions
  csu_lan_landed_state_determination : csu_lan_landed_state_determination_lib/csu_lan_landed_state_determination
  vector_magnitude : util_common_lib/vector_magnitude  SystemSampleTime=-1
  lander_state_bus : Outport
  wires:
  Switch1/1 -> [landed]
  actuator_torques/1 -> csc_eom_six_dof_integration_fwdeuler/2(actuator_torques)
  ext_force/1 -> csc_kin_kinematic_propagation/4, csc_eom_six_dof_integration_fwdeuler/3(external_forces_torques), Bus Selector1/1
  [time] -> csc_eom_six_dof_integration_fwdeuler/11(time)
  Data Type Conversion/1 -> Switch1/3, Logical Operator2/1
  Unit Delay2/1 -> Data Type Conversion/1
  Constant/1 -> Switch1/1
  Logical Operator2/1 -> Switch1/2
  [landed] -> csu_ini_initial_conditions/1
  Switch/1 -> Bus Selector/1, lander_state_bus/1
  time/1 -> [time]  "clock"
  csu_ini_initial_conditions/1 -> csc_eom_six_dof_integration_fwdeuler/7(initial_velocity_I)
  csu_ini_initial_conditions/2 -> csc_eom_six_dof_integration_fwdeuler/8(initial_position_I)
  csu_ini_initial_conditions/3 -> csc_eom_six_dof_integration_fwdeuler/9(initial_rate_body_eci_B)
  csu_ini_initial_conditions/4 -> csc_eom_six_dof_integration_fwdeuler/10(initial_q_body_from_eci)
  inertia_tensor/1 -> csc_eom_six_dof_integration_fwdeuler/4(inertia_tensor)
  Constant7/1 -> csc_eom_six_dof_integration_fwdeuler/6(integrator_reset)
  mass/1 -> csc_eom_six_dof_integration_fwdeuler/5(mass), Product1/2
  actuator_forces_B/1 -> [thrust], csc_eom_six_dof_integration_fwdeuler/1(actuator_forces_B)
  [time] -> csc_kin_kinematic_propagation/1
  [landed] -> csc_kin_kinematic_propagation/Enable
  [landed] -> Logical Operator/1
  [landed] -> Switch/2
  [time] -> csu_lan_landed_state_determination/1
  Bus Selector/1 -> csu_lan_landed_state_determination/2  "<rtk_pos_eci>"
  Bus Selector/2 -> csu_lan_landed_state_determination/3  "<rrk_q_body_from_eci>"
  [landed] -> csu_lan_landed_state_determination/4
  csu_lan_landed_state_determination/3 -> Unit Delay2/1
  Logical Operator/1 -> csc_eom_six_dof_integration_fwdeuler/Enable
  Bus Selector1/1 -> vector_magnitude/1  "<grav_acc_inertial>"
  Selector/1 -> Product2/1, Compare To Constant/1
  vector_magnitude/1 -> Product1/1
  Product1/1 -> Product2/2
  Compare To Constant/1 -> Logical Operator2/2
  Compare To Constant1/1 -> Logical Operator2/4
  Product2/1 -> Compare To Constant1/1
  csc_eom_six_dof_integration_fwdeuler/1(ballistic_state) -> Switch/3
  csc_kin_kinematic_propagation/1 -> Switch/1
  csu_lan_landed_state_determination/1 -> Unit Delay4/1
  csu_lan_landed_state_determination/2 -> Unit Delay3/1
  state_in/1 -> Bus Selector2/1, csu_ini_initial_conditions/2
  Unit Delay3/1 -> csc_kin_kinematic_propagation/3
  Unit Delay4/1 -> csc_kin_kinematic_propagation/2
  [thrust] -> Selector/1
  Bus Selector2/2 -> J2000 to MCMF Velocity Transformation Quaternion1/3  "<rtk_vel_eci>"
  MCMF to Topocentric Transformation Quaternion/2 -> Selector1/1
  Selector1/1 -> [z_vel]
  [z_vel] -> Compare To Constant2/1
  Compare To Constant2/1 -> Logical Operator2/3
  J2000 to MCMF Velocity Transformation Quaternion1/2 -> MCMF to Topocentric Transformation Quaternion/1
  MCMF to Topocentric Transformation Quaternion/1 -> Terminator/1
  J2000 to MCMF Velocity Transformation Quaternion1/1 -> Terminator1/1
  [time] -> J2000 to MCMF Velocity Transformation Quaternion1/1
  Bus Selector2/1 -> J2000 to MCMF Velocity Transformation Quaternion1/2  "<rtk_pos_eci>"

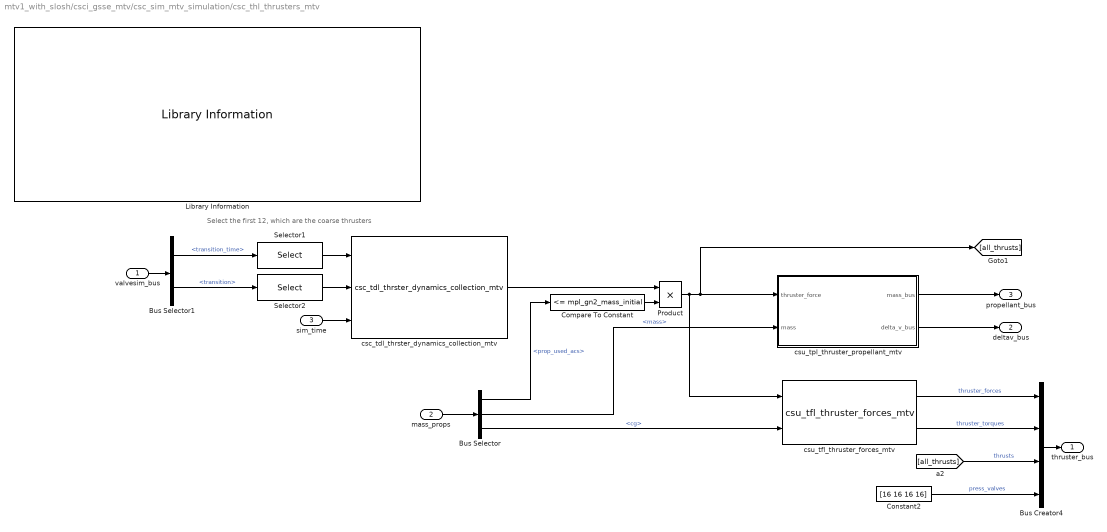
== system mtv1_with_slosh/csci_gsse_mtv/csc_sim_mtv_simulation/csc_thl_thrusters_mtv ==
  note: Select the first 12, which are the coarse thrusters
  valvesim_bus : Inport
  mass_props : Inport  Port=2
  sim_time : Inport  Port=3
  Bus Creator4 : BusCreator  OutDataTypeStr=Bus: actuator_mtv_msg_t
  Bus Selector : BusSelector  OutputSignals=prop_used_acs,mass,cg
  Bus Selector1 : BusSelector  OutputSignals=transition_time,transition
  Compare To Constant : simulink/Logic and Bit Operations/Compare To Constant  relop=<=  const=mpl_gn2_mass_initial  OutDataTypeStr=uint8
  Constant2 : Constant  Value=[16 16 16 16]  OutDataTypeStr=uint8
  Library Information : util_info_lib/Library Information  owner='NONE'
  Product : Product
  Selector1 : Selector  InputPortWidth=22  Indices=[1:12]
  Selector2 : Selector  InputPortWidth=22  Indices=[1:12]
  csc_tdl_thrster_dynamics_collection_mtv : csc_tdl_thruster_dynamics_collection_mtv_lib/csc_tdl_thrster_dynamics_collection_mtv  SystemSampleTime=-1
  csu_tfl_thruster_forces_mtv : csu_tfl_thruster_forces_mtv_lib/csu_tfl_thruster_forces_mtv
  csu_tpl_thruster_propellant_mtv : Subsystem  AncestorBlock=csu_tpl_thruster_propellant_mtv_lib/csu_tpl_thruster_propellant_mtv
  thruster_bus : Outport
  deltav_bus : Outport  Port=2
  propellant_bus : Outport  Port=3
  wires:
  Product/1 -> csu_tfl_thruster_forces_mtv/1, [all_thrusts], csu_tpl_thruster_propellant_mtv/1(thruster_force)
  mass_props/1 -> Bus Selector/1
  Bus Selector/2 -> csu_tpl_thruster_propellant_mtv/2(mass)  "<mass>"
  Bus Selector/3 -> csu_tfl_thruster_forces_mtv/2  "<cg>"
  sim_time/1 -> csc_tdl_thrster_dynamics_collection_mtv/3
  valvesim_bus/1 -> Bus Selector1/1
  csu_tpl_thruster_propellant_mtv/2(delta_v_bus) -> deltav_bus/1
  csu_tpl_thruster_propellant_mtv/1(mass_bus) -> propellant_bus/1
  Bus Selector1/2 -> Selector2/1  "<transition>"
  Bus Selector1/1 -> Selector1/1  "<transition_time>"
  Bus Creator4/1 -> thruster_bus/1
  csu_tfl_thruster_forces_mtv/2 -> Bus Creator4/2  "thruster_torques"
  csu_tfl_thruster_forces_mtv/1 -> Bus Creator4/1  "thruster_forces"
  [all_thrusts] -> Bus Creator4/3  "thrusts"
  csc_tdl_thrster_dynamics_collection_mtv/1 -> Product/1
  Compare To Constant/1 -> Product/2
  Selector1/1 -> csc_tdl_thrster_dynamics_collection_mtv/1
  Selector2/1 -> csc_tdl_thrster_dynamics_collection_mtv/2
  Bus Selector/1 -> Compare To Constant/1  "<prop_used_acs>"
  Constant2/1 -> Bus Creator4/4  "press_valves"

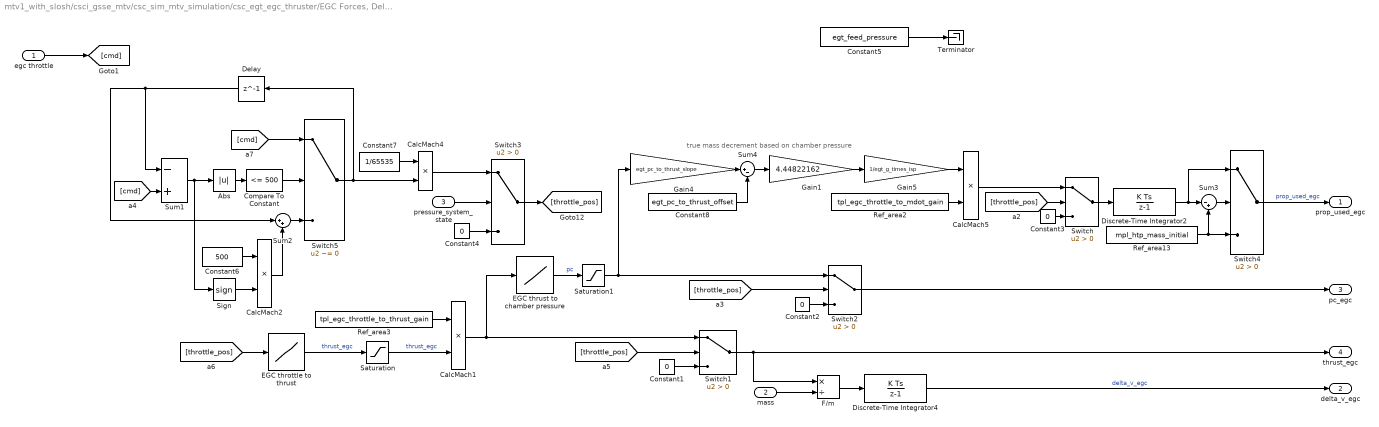
== system mtv1_with_slosh/csci_gsse_mtv/csc_sim_mtv_simulation/csc_egt_egc_thruster/EGC Forces, Delta-V and Propellant Usage ==
  note: true mass decrement based on chamber pressure
  egc throttle : Inport
  mass : Inport  Port=2
  pressure_system_state : Inport  Port=3
  Abs : Abs
  CalcMach{1..2,4..5} (4 alike) : Product  SaturateOnIntegerOverflow=on  OutDataTypeStr=Inherit: Same as first input
  Compare To Constant : simulink/Logic and Bit Operations/Compare To Constant  relop=<=  const=500  OutDataTypeStr=boolean
  Constant{1..4} (4 alike) : Constant  Value=0
  Constant5 : Constant  Value=egt_feed_pressure
  Constant6 : Constant  Value=500
  Constant7 : Constant  Value=1/65535
  Constant8 : Constant  Value=egt_pc_to_thrust_offset  OutDataTypeStr=double
  Delay : Delay  DelayLength=1
  Discrete-Time Integrator2 : DiscreteIntegrator  gainval=1  SampleTime=sim_time_step_size
  Discrete-Time Integrator4 : DiscreteIntegrator  gainval=1  SampleTime=sim_time_step_size
  "EGC thrust to chamber pressure " : Lookup  InputValues=tpl_egc_chamber_pressure_to_thrust(:,2)  Table=tpl_egc_chamber_pressure_to_thrust(:,1)
  EGC throttle to thrust : Lookup  InputValues=tpl_egc_throttle_to_thrust(:,1)  Table=tpl_egc_throttle_to_thrust(:,2)
  F/m : Product  Inputs=*/
  Gain1 : Gain  Gain=4.44822162
  Gain4 : Gain  Gain=egt_pc_to_thrust_slope
  Gain5 : Gain  Gain=1/egt_g_times_isp
  Ref_area13 : Constant  Value=mpl_htp_mass_initial
  Ref_area2 : Constant  Value=tpl_egc_throttle_to_mdot_gain
  Ref_area3 : Constant  Value=tpl_egc_throttle_to_thrust_gain
  Saturation : Saturate  UpperLimit=2300  LowerLimit=0
  Saturation1 : Saturate  UpperLimit=600  LowerLimit=0
  Sign : Signum
  Sum1 : Sum  Inputs=-+
  Sum2 : Sum  Inputs=|++
  Sum3 : Sum  Inputs=|-+
  Sum4 : Sum  Inputs=|+-
  Switch{,1..4} (5 alike) : Switch  Criteria=u2 > Threshold
  Switch5 : Switch  Criteria=u2 ~= 0
  Terminator : Terminator
  prop_used_egc : Outport
  delta_v_egc : Outport  Port=2
  pc_egc : Outport  Port=3
  thrust_egc : Outport  Port=4
  wires:
  CalcMach1/1 -> Switch1/1, "EGC thrust to chamber pressure "/1
  Switch2/1 -> pc_egc/1
  [throttle_pos] -> Switch2/2
  Constant2/1 -> Switch2/3
  Saturation/1 -> CalcMach1/2  "thrust_egc"
  [throttle_pos] -> Switch1/2
  Constant1/1 -> Switch1/3
  Switch1/1 -> F/m/1, thrust_egc/1
  Switch/1 -> Discrete-Time Integrator2/1
  [throttle_pos] -> Switch/2
  Constant3/1 -> Switch/3
  mass/1 -> F/m/2
  F/m/1 -> Discrete-Time Integrator4/1
  Switch4/1 -> prop_used_egc/1  "prop_used_egc"
  Discrete-Time Integrator4/1 -> delta_v_egc/1  "delta_v_egc"
  pressure_system_state/1 -> Switch3/2
  Constant4/1 -> Switch3/3
  Sum3/1 -> Switch4/2
  Discrete-Time Integrator2/1 -> Switch4/1, Sum3/1
  Ref_area13/1 -> Switch4/3, Sum3/2
  Constant5/1 -> Terminator/1
  Gain5/1 -> CalcMach5/1
  Ref_area3/1 -> CalcMach1/1
  egc throttle/1 -> [cmd]
  Delay/1 -> Sum1/1, Sum2/1
  Sum1/1 -> Sign/1, Abs/1
  Abs/1 -> Compare To Constant/1
  Compare To Constant/1 -> Switch5/2
  [cmd] -> Sum1/2
  [cmd] -> Switch5/1
  Switch5/1 -> CalcMach4/2, Delay/1
  Sum2/1 -> Switch5/3
  CalcMach2/1 -> Sum2/2
  Constant6/1 -> CalcMach2/1
  Sign/1 -> CalcMach2/2
  CalcMach4/1 -> Switch3/1
  Constant7/1 -> CalcMach4/1
  "EGC thrust to chamber pressure "/1 -> Saturation1/1  "pc"
  Sum4/1 -> Gain1/1
  Gain1/1 -> Gain5/1
  Gain4/1 -> Sum4/1
  Constant8/1 -> Sum4/2
  Switch3/1 -> [throttle_pos]
  [throttle_pos] -> EGC throttle to thrust/1
  EGC throttle to thrust/1 -> Saturation/1  "thrust_egc"
  Saturation1/1 -> Switch2/1, Gain4/1
  Ref_area2/1 -> CalcMach5/2
  CalcMach5/1 -> Switch/1

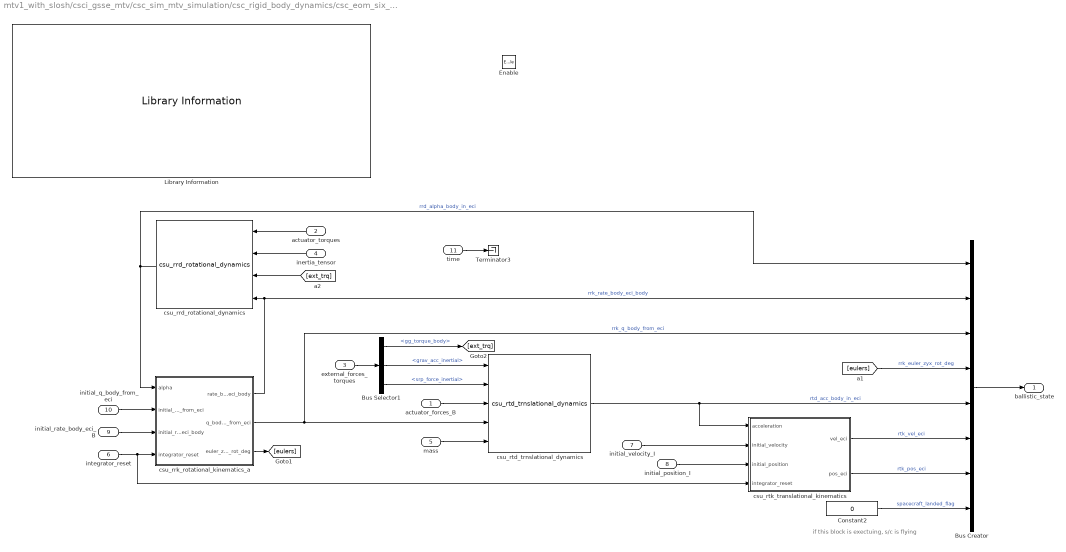
== system mtv1_with_slosh/csci_gsse_mtv/csc_sim_mtv_simulation/csc_rigid_body_dynamics/csc_eom_six_dof_integration_fwdeuler ==
  note: if this block is exectuing, s/c is flying
  actuator_forces_B : Inport
  actuator_torques : Inport  Port=2
  external_forces_torques : Inport  Port=3
  inertia_tensor : Inport  Port=4
  mass : Inport  Port=5
  integrator_reset : Inport  Port=6
  initial_velocity_I : Inport  Port=7
  initial_position_I : Inport  Port=8
  initial_rate_body_eci_B : Inport  Port=9
  initial_q_body_from_eci : Inport  Port=10
  time : Inport  Port=11
  Enable : EnablePort  StatesWhenEnabling=reset
  Bus Creator : BusCreator  Inputs=8  OutDataTypeStr=Bus: lander_state_bus_t
  Bus Selector1 : BusSelector  OutputSignals=gg_torque_body,grav_acc_inertial,srp_force_inertial
  Constant2 : Constant  Value=0
  Library Information : util_info_lib/Library Information  owner='escrane'
  Terminator3 : Terminator
  csu_rrd_rotational_dynamics : csu_rrd_rotational_dynamics_lib/csu_rrd_rotational_dynamics
  csu_rrk_rotational_kinematics_a : Subsystem  AncestorBlock=csu_rrk_rotational_kinematics_lib/csu_rrk_rotational_kinematics
  csu_rtd_trnslational_dynamics : csu_rtd_translational_dynamics_lib/csu_rtd_trnslational_dynamics
  csu_rtk_translational_kinematics : Subsystem  AncestorBlock=csu_rtk_translational_kinematics_lib/csu_rtk_translational_kinematics
  ballistic_state : Outport
  wires:
  time/1 -> Terminator3/1
  actuator_torques/1 -> csu_rrd_rotational_dynamics/1
  inertia_tensor/1 -> csu_rrd_rotational_dynamics/2
  initial_q_body_from_eci/1 -> csu_rrk_rotational_kinematics_a/2(initial_q_body_from_eci)
  initial_rate_body_eci_B/1 -> csu_rrk_rotational_kinematics_a/3(initial_rate_body_eci_body)
  integrator_reset/1 -> csu_rrk_rotational_kinematics_a/4(integrator_reset), csu_rtk_translational_kinematics/4(integrator_reset)
  mass/1 -> csu_rtd_trnslational_dynamics/5
  actuator_forces_B/1 -> csu_rtd_trnslational_dynamics/3
  initial_velocity_I/1 -> csu_rtk_translational_kinematics/2(initial_velocity)
  initial_position_I/1 -> csu_rtk_translational_kinematics/3(initial_position)
  csu_rrk_rotational_kinematics_a/3(euler_zyx_rot_deg) -> [eulers]
  csu_rtk_translational_kinematics/2(pos_eci) -> Bus Creator/7  "rtk_pos_eci"
  csu_rtk_translational_kinematics/1(vel_eci) -> Bus Creator/6  "rtk_vel_eci"
  csu_rtd_trnslational_dynamics/1 -> csu_rtk_translational_kinematics/1(acceleration), Bus Creator/5  "rtd_acc_body_in_eci"
  csu_rrk_rotational_kinematics_a/1(rate_body_eci_body) -> csu_rrd_rotational_dynamics/4, Bus Creator/2  "rrk_rate_body_eci_body"
  [eulers] -> Bus Creator/4  "rrk_euler_zyx_rot_deg"
  csu_rrd_rotational_dynamics/1 -> csu_rrk_rotational_kinematics_a/1(alpha), Bus Creator/1  "rrd_alpha_body_in_eci"
  csu_rrk_rotational_kinematics_a/2(q_body_from_eci) -> Bus Creator/3, csu_rtd_trnslational_dynamics/4  "rrk_q_body_from_eci"
  Bus Creator/1 -> ballistic_state/1
  external_forces_torques/1 -> Bus Selector1/1
  Bus Selector1/3 -> csu_rtd_trnslational_dynamics/2  "<srp_force_inertial>"
  Bus Selector1/1 -> [ext_trq]  "<gg_torque_body>"
  Bus Selector1/2 -> csu_rtd_trnslational_dynamics/1  "<grav_acc_inertial>"
  [ext_trq] -> csu_rrd_rotational_dynamics/3
  Constant2/1 -> Bus Creator/8  "spacecraft_landed_flag"

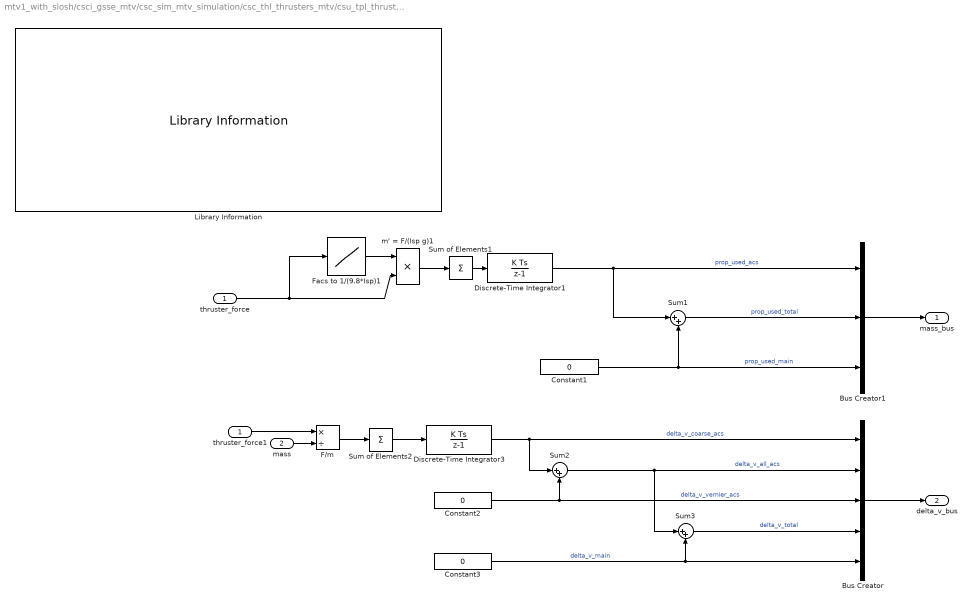
== system mtv1_with_slosh/csci_gsse_mtv/csc_sim_mtv_simulation/csc_thl_thrusters_mtv/csu_tpl_thruster_propellant_mtv ==
  thruster_force : Inport
  mass : Inport  Port=2
  Bus Creator : BusCreator  Inputs=5
  Bus Creator1 : BusCreator  Inputs=3
  Constant1 : Constant  Value=0  OutDataTypeStr=double
  Constant2 : Constant  Value=0  OutDataTypeStr=double
  Constant3 : Constant  Value=0  OutDataTypeStr=double
  Discrete-Time Integrator1 : DiscreteIntegrator  gainval=1  SampleTime=sim_time_step_size
  Discrete-Time Integrator3 : DiscreteIntegrator  gainval=1  SampleTime=sim_time_step_size
  F/m : Product  Inputs=*/
  Facs to 1/(9.8*Isp)1 : Lookup  InputValues=tpl_coarse_acs_thrust_to_isp(:,1)  Table=1./(9.8*tpl_coarse_acs_thrust_to_isp(:,2))  LookUpMeth=Interpolation-Use End Values
  Library Information : util_info_lib/Library Information  owner='escrane'
  Sum of Elements1 : Sum  Inputs=+
  Sum of Elements2 : Sum  Inputs=+
  Sum1 : Sum  Inputs=|++
  Sum2 : Sum  Inputs=|++
  Sum3 : Sum  Inputs=|++
  m' = F/(Isp g)1 : Product  RndMeth=Zero
  thruster_force1 : InportShadow
  mass_bus : Outport
  delta_v_bus : Outport  Port=2
  wires:
  Sum2/1 -> Sum3/1, Bus Creator/2  "delta_v_all_acs"
  Discrete-Time Integrator3/1 -> Sum2/1, Bus Creator/1  "delta_v_coarse_acs"
  Constant2/1 -> Sum2/2, Bus Creator/3  "delta_v_vernier_acs"
  Discrete-Time Integrator1/1 -> Sum1/1, Bus Creator1/1  "prop_used_acs"
  Sum1/1 -> Bus Creator1/2  "prop_used_total"
  m' = F/(Isp g)1/1 -> Sum of Elements1/1
  Facs to 1/(9.8*Isp)1/1 -> m' = F/(Isp g)1/1
  thruster_force/1 -> Facs to 1/(9.8*Isp)1/1, m' = F/(Isp g)1/2
  Sum of Elements1/1 -> Discrete-Time Integrator1/1
  Constant1/1 -> Sum1/2, Bus Creator1/3  "prop_used_main"
  mass/1 -> F/m/2
  F/m/1 -> Sum of Elements2/1
  Sum of Elements2/1 -> Discrete-Time Integrator3/1
  Sum3/1 -> Bus Creator/4  "delta_v_total"
  Constant3/1 -> Sum3/2, Bus Creator/5  "delta_v_main"
  Bus Creator/1 -> delta_v_bus/1
  Bus Creator1/1 -> mass_bus/1
  thruster_force1/1 -> F/m/1

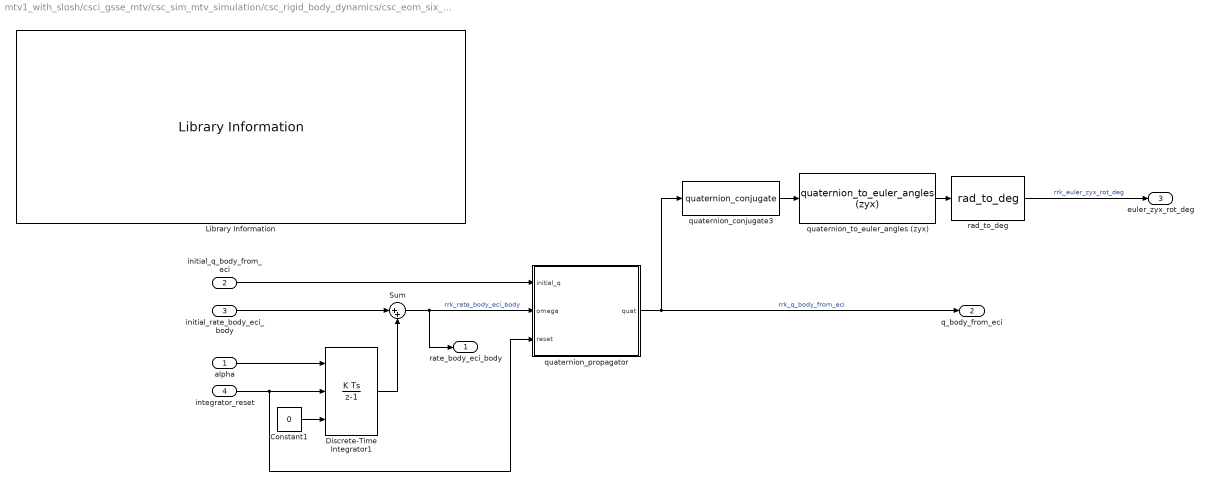
== system mtv1_with_slosh/csci_gsse_mtv/csc_sim_mtv_simulation/csc_rigid_body_dynamics/csc_eom_six_dof_integration_fwdeuler/csu_rrk_rotational_kinematics_a ==
  alpha : Inport
  initial_q_body_from_eci : Inport  Port=2
  initial_rate_body_eci_body : Inport  Port=3
  integrator_reset : Inport  Port=4
  Constant1 : Constant  Value=0
  Discrete-Time Integrator1 : DiscreteIntegrator  ExternalReset=rising  InitialConditionSource=external  InitialConditionSetting=State (most efficient)  SampleTime=sim_time_step_size
  Library Information : util_info_lib/Library Information  owner='NONE'
  Sum : Sum  Inputs=|++
  quaternion_conjugate3 : util_quat_lib/quaternion_conjugate  SystemSampleTime=-1
  quaternion_propagator : Subsystem  AncestorBlock=util_quat_lib/quaternion_propagator
      mask Display:
      | disp('propogate(q)')
      | color('blue')
      | text(0.05,0.02,'NASA',...
      |  	'HorizontalAlignment','Left',...
      | 	'VerticalAlignment','bottom')
  quaternion_to_euler_angles (zyx) : util_quat_lib/quaternion_to_euler_angles (zyx)  SystemSampleTime=-1
  rad_to_deg : util_common_lib/rad_to_deg  SystemSampleTime=-1
  rate_body_eci_body : Outport
  q_body_from_eci : Outport  Port=2
  euler_zyx_rot_deg : Outport  Port=3
  wires:
  quaternion_propagator/1(quat) -> quaternion_conjugate3/1, q_body_from_eci/1  "rrk_q_body_from_eci"
  integrator_reset/1 -> quaternion_propagator/3(reset), Discrete-Time Integrator1/2
  Constant1/1 -> Discrete-Time Integrator1/3
  alpha/1 -> Discrete-Time Integrator1/1
  initial_rate_body_eci_body/1 -> Sum/1
  Discrete-Time Integrator1/1 -> Sum/2
  Sum/1 -> quaternion_propagator/2(omega), rate_body_eci_body/1  "rrk_rate_body_eci_body"
  initial_q_body_from_eci/1 -> quaternion_propagator/1(initial_q)
  quaternion_to_euler_angles (zyx)/1 -> rad_to_deg/1
  rad_to_deg/1 -> euler_zyx_rot_deg/1  "rrk_euler_zyx_rot_deg"
  quaternion_conjugate3/1 -> quaternion_to_euler_angles (zyx)/1

== system mtv1_with_slosh/csci_gsse_mtv/csc_sim_mtv_simulation/csc_rigid_body_dynamics/csc_eom_six_dof_integration_fwdeuler/csu_rtk_translational_kinematics ==
  acceleration : Inport
  initial_velocity : Inport  Port=2
  initial_position : Inport  Port=3
  integrator_reset : Inport  Port=4
  Constant1 : Constant  Value=0
  Constant2 : Constant  Value=0
  Discrete-Time Integrator1 : DiscreteIntegrator  ExternalReset=rising  InitialConditionSource=external  InitialConditionSetting=State (most efficient)  SampleTime=sim_time_step_size
  Discrete-Time Integrator2 : DiscreteIntegrator  ExternalReset=rising  InitialConditionSource=external  InitialConditionSetting=State (most efficient)  SampleTime=sim_time_step_size
  Library Information : util_info_lib/Library Information  owner='NONE'
  Sum : Sum  Inputs=++|
  Sum1 : Sum  Inputs=|++
  vel_eci : Outport
  pos_eci : Outport  Port=2
  wires:
  initial_position/1 -> Sum1/2
  Sum1/1 -> pos_eci/1  "rtk_pos_eci"
  Constant1/1 -> Discrete-Time Integrator2/3
  Sum/1 -> Discrete-Time Integrator2/1, vel_eci/1  "rtk_vel_eci"
  acceleration/1 -> Discrete-Time Integrator1/1
  Constant2/1 -> Discrete-Time Integrator1/3
  initial_velocity/1 -> Sum/1
  Discrete-Time Integrator2/1 -> Sum1/1
  Discrete-Time Integrator1/1 -> Sum/2
  integrator_reset/1 -> Discrete-Time Integrator2/2, Discrete-Time Integrator1/2
